simulink model "AirCtl_Co"  (R2016b)
settings: configuration reference "CodeGenConfigSet" (kept outside this file)
values from neighbouring files (symbols this model uses):
  AirCtl_swtTypCor_C = Calibration.Parameter    [init_AirCtl_Co.m]    (also in init_AirCtl_Co_SIL.m = Simulink.Parameter)
  INJ_MASS_ZERO = fi(0,FuelMass_mg_hub)    [init_AirCtl_Co.m]    (also in init_AirCtl_Co_SIL.m)
  TRQ_ZERO = fi(0,Trq_Nm)    [init_AirCtl_Co.m]    (also in init_AirCtl_Co_SIL.m)
settings Model: Creator=Wollf  LastModifiedBy=zhulinfeng
settings ConfigSetRef: SourceLocation=Base Workspace

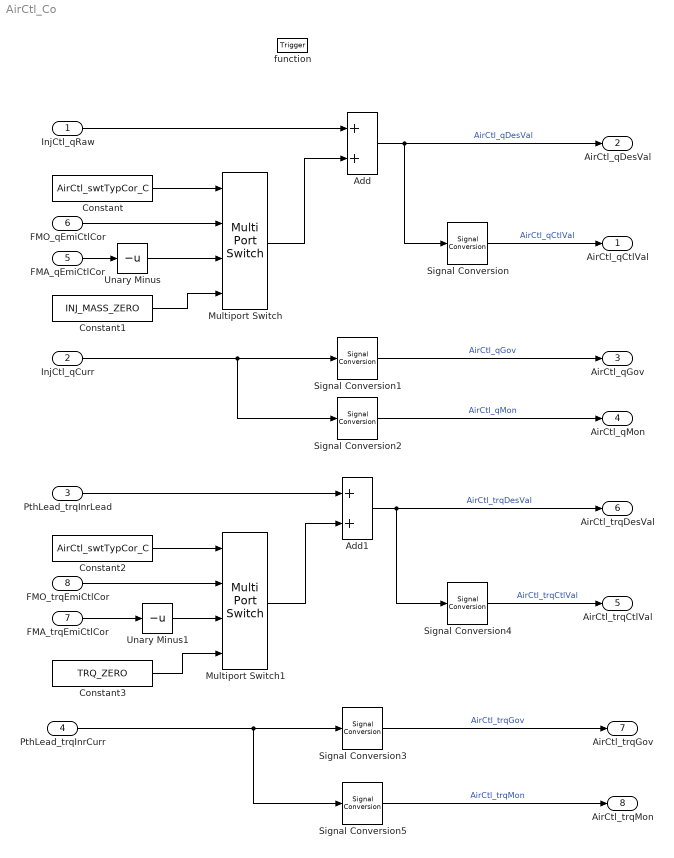
== system AirCtl_Co ==
  InjCtl_qRaw : Inport  Tag=mg/hub  Description=Raw value of injection mass  OutMin=-319  OutMax=319  OutDataTypeStr=FuelMass_mg_hub
  InjCtl_qCurr : Inport  Tag=mg/hub  Description=Torque generating engine fuel injection quantity  Port=2  OutMin=-319  OutMax=319  OutDataTypeStr=FuelMass_mg_hub
  PthLead_trqInrLead : Inport  Tag=Nm  Description=Inner torque lead value  Port=3  OutMin=-3000  OutMax=3000  OutDataTypeStr=Trq_Nm
  PthLead_trqInrCurr : Inport  Tag=Nm  Description=Actual percent engine torque  Port=4  OutMin=-3000  OutMax=3000  OutDataTypeStr=Trq_Nm
  FMA_qEmiCtlCor : Inport  Tag=mg/hub  Description=FMA fuel mass correction quantity for emission control  Port=5  OutMin=-319  OutMax=319  OutDataTypeStr=FuelMass_mg_hub
  FMO_qEmiCtlCor : Inport  Tag=mg/hub  Description=FMO correction quantity for emission control  Port=6  OutMin=-319  OutMax=319  OutDataTypeStr=FuelMass_mg_hub
  FMA_trqEmiCtlCor : Inport  Tag=Nm  Description=FMA torque correction quantity for emission control  Port=7  OutMin=-3000  OutMax=3000  OutDataTypeStr=Trq_Nm
  FMO_trqEmiCtlCor : Inport  Tag=Nm  Description=FMO torque correction for emission control  Port=8  OutMin=-3000  OutMax=3000  OutDataTypeStr=Trq_Nm
  function : TriggerPort  TriggerType=function-call  VariantControl=Variant
  Add : Sum  SaturateOnIntegerOverflow=on  InputSameDT=on
  Add1 : Sum  SaturateOnIntegerOverflow=on  InputSameDT=on
  Constant : Constant  Value=AirCtl_swtTypCor_C
  Constant1 : Constant  Value=INJ_MASS_ZERO  OutDataTypeStr=Inherit: Inherit via back propagation
  Constant2 : Constant  Value=AirCtl_swtTypCor_C
  Constant3 : Constant  Value=TRQ_ZERO  OutDataTypeStr=Inherit: Inherit via back propagation
  Multiport Switch : MultiPortSwitch  DataPortOrder=Specify indices  DataPortIndices={1,2,0}  InputSameDT=on
  Multiport Switch1 : MultiPortSwitch  DataPortOrder=Specify indices  DataPortIndices={1,2,0}  InputSameDT=on
  Signal Conversion{,1..5} (6 alike) : SignalConversion  OverrideOpt=off
  Unary Minus : UnaryMinus
  Unary Minus1 : UnaryMinus
  AirCtl_qCtlVal : Outport  Tag=mg/hub  Description=Injection quantity for the open-loop control of the exhaust-gas recirculation control  OutMin=-300  OutMax=300  OutDataTypeStr=FuelMass_mg_hub
  AirCtl_qDesVal : Outport  Tag=mg/hub  Description=Inner quantity for open-loop control of the exhaustgas recirculation control  Port=2  OutMin=-300  OutMax=300  OutDataTypeStr=FuelMass_mg_hub
  AirCtl_qGov : Outport  Tag=mg/hub  Description=Inner quantity for open-loop control of the exhaustgas recirculation control  Port=3  OutMin=-300  OutMax=300  OutDataTypeStr=FuelMass_mg_hub
  AirCtl_qMon : Outport  Tag=mg/hub  Description=Inner quantity of monitoring level for open-loop control of the exhaustgas recirculation control  Port=4  OutMin=-300  OutMax=300  OutDataTypeStr=FuelMass_mg_hub
  AirCtl_trqCtlVal : Outport  Tag=Nm  Description=Injection torque for the open-loop control of the exhaust-gas recirculation control  Port=5  OutMin=-3000  OutMax=3000  OutDataTypeStr=Trq_Nm
  AirCtl_trqDesVal : Outport  Tag=Nm  Description=Inner torque for open-loop control of the exhaustgas recirculation control  Port=6  OutMin=-3000  OutMax=3000  OutDataTypeStr=Trq_Nm
  AirCtl_trqGov : Outport  Tag=Nm  Description=Inner torque for open-loop control of the exhaustgas recirculation control  Port=7  OutMin=-3000  OutMax=3000  OutDataTypeStr=Trq_Nm
  AirCtl_trqMon : Outport  Tag=Nm  Description=Inner torque of monitoring level for open-loop control of the exhaustgas recirculation control  Port=8  OutMin=-3000  OutMax=3000  OutDataTypeStr=Trq_Nm
  wires:
  Signal Conversion/1 -> AirCtl_qCtlVal/1  "AirCtl_qCtlVal"
  Add/1 -> AirCtl_qDesVal/1, Signal Conversion/1  "AirCtl_qDesVal"
  Signal Conversion1/1 -> AirCtl_qGov/1  "AirCtl_qGov"
  Signal Conversion2/1 -> AirCtl_qMon/1  "AirCtl_qMon"
  Signal Conversion4/1 -> AirCtl_trqCtlVal/1  "AirCtl_trqCtlVal"
  Add1/1 -> Signal Conversion4/1, AirCtl_trqDesVal/1  "AirCtl_trqDesVal"
  Signal Conversion3/1 -> AirCtl_trqGov/1  "AirCtl_trqGov"
  Signal Conversion5/1 -> AirCtl_trqMon/1  "AirCtl_trqMon"
  InjCtl_qRaw/1 -> Add/1
  Multiport Switch/1 -> Add/2
  FMO_qEmiCtlCor/1 -> Multiport Switch/2
  FMA_qEmiCtlCor/1 -> Unary Minus/1
  Constant/1 -> Multiport Switch/1
  Constant1/1 -> Multiport Switch/4
  Unary Minus/1 -> Multiport Switch/3
  InjCtl_qCurr/1 -> Signal Conversion2/1, Signal Conversion1/1
  PthLead_trqInrLead/1 -> Add1/1
  Constant2/1 -> Multiport Switch1/1
  Unary Minus1/1 -> Multiport Switch1/3
  Constant3/1 -> Multiport Switch1/4
  Multiport Switch1/1 -> Add1/2
  PthLead_trqInrCurr/1 -> Signal Conversion5/1, Signal Conversion3/1
  FMA_trqEmiCtlCor/1 -> Unary Minus1/1
  FMO_trqEmiCtlCor/1 -> Multiport Switch1/2
